simulink model "test_birdseye_transform"  (R2019a)
settings: Solver=VariableStepAuto  StartTime=0.0  StopTime=1  RelTol=1e-3
values from neighbouring files (symbols this model uses):
  T_unreal = tform.T    [estimate_birdseye_transform.m]
undefined symbols (not defined in the file or in its folder): gray, Rec, SDTV
libraries: visiongeotforms x2, visionhdlio x2, visionhdlgeotforms x1, visionconversions x1, visionsources x1, visionhdlutilities x1
settings Model: Creator=tstraessle  LastModifiedBy=timo.straessle

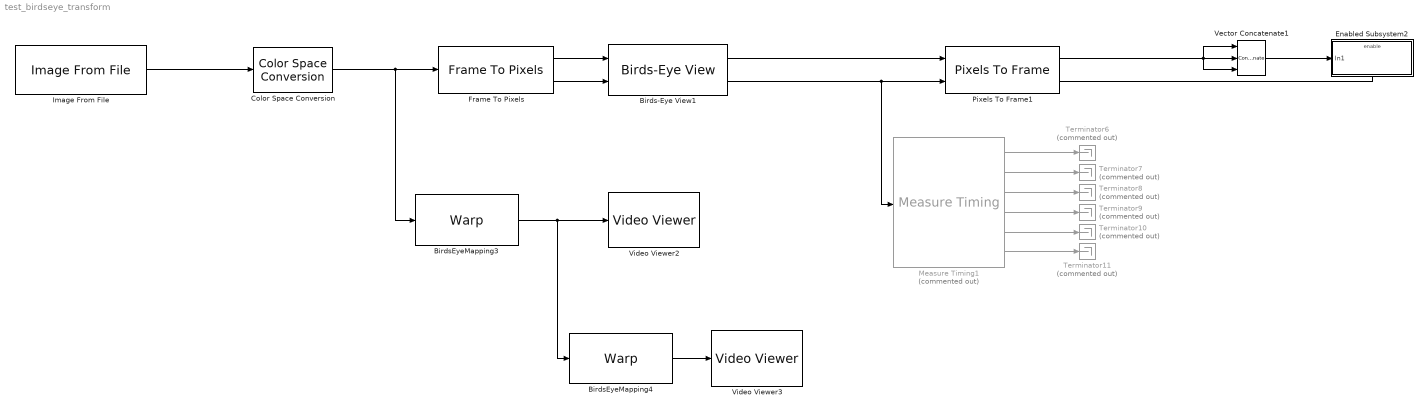
== system test_birdseye_transform ==
  Birds-Eye View1 : visionhdlgeotforms/Birds-Eye View  HomographyMatrix=T_unreal  MaxBufferSize=200000*2  MaxSourceLinesBuffered=100*2  BirdsEyeActivePixels=1920  BirdsEyeActiveLines=1080  SimulateUsing=Code generation
      settings: SourceProductName=Vision HDL Toolbox  SourceProductBaseCode=VT
  BirdsEyeMapping3 : visiongeotforms/Warp  TransformMatrixSource=Custom  TransformMatrix=T_unreal  InterpolationMethod=Bilinear  BackgroundFillValue=0  OutputImagePositionSource=Custom  OutputImagePosition=[ 1, 1, 1920, 1080 ]  ROIInputPort=off  ROIValidityOutputPort=off  SimulateUsing=Code generation
      settings: SourceProductName=Computer Vision Toolbox  SourceProductBaseCode=VP
  BirdsEyeMapping4 : visiongeotforms/Warp  TransformMatrixSource=Custom  TransformMatrix=inv(T_unreal)  InterpolationMethod=Bilinear  BackgroundFillValue=0  OutputImagePositionSource=Custom  OutputImagePosition=[ 1, 1, 1920, 1080 ]  ROIInputPort=off  ROIValidityOutputPort=off  SimulateUsing=Code generation
      settings: SourceProductName=Computer Vision Toolbox  SourceProductBaseCode=VP
  Color Space Conversion : visionconversions/Color Space  Conversion  conversion=Obsolete  conversionActive=R'G'B' to intensity  wp_str=D65  rec=Rec. 601 (SDTV)  sys=1125/60/2:1  imagePorts=One multidimensional signal
  Enabled Subsystem2 : Subsystem  TreatAsAtomicUnit=on
  Frame To Pixels : visionhdlio/Frame To Pixels  NumComponents=1  VideoFormat=1080p  ActivePixelsPerLine=1280  ActiveVideoLines=720  TotalPixelsPerLine=1650  TotalVideoLines=1100  StartingActiveLine=25  FrontPorch=110  SampleTime=0
      settings: SourceProductName=Vision HDL Toolbox  SourceProductBaseCode=VT
  Image From File : visionsources/Image From File  Tag=vipblks_nd  FileName=C:\SVN\AE\content_creation\demos\ID83 - Lane Detection on FPGA\new version\support files\images\snapshot_straight_road.bmp  Ts=1/60  imagePorts=One multidimensional signal  OutPortLabels=R|G|B  ImageDataType=uint8  sdImageDataType=uint(8)  Signed=on  WordLength=16  FractionLengthMode=User-defined  FractionLength=15
      settings: SourceProductName=Computer Vision Toolbox
  Measure Timing1 : visionhdlutilities/Measure Timing  Commented=on  SimulateUsing=Code generation
      settings: SourceProductName=Vision HDL Toolbox  SourceProductBaseCode=VT
  Pixels To Frame1 : visionhdlio/Pixels To Frame  NumComponents=1  VideoFormat=1080p  ActivePixelsPerLine=1280  ActiveVideoLines=1050  TotalPixelsPerLine=1650  TotalVideoLines=1100
      settings: SourceProductName=Vision HDL Toolbox  SourceProductBaseCode=VT
  Terminator{6..11} (6 alike) : Terminator  Commented=on
  Vector Concatenate1 : Concatenate  NumInputs=3  Mode=Multidimensional array  ConcatenateDimension=3
  Video Viewer2 : VideoViewer  colormapValue=gray(256)  FigPos=[1105 1039 769 647]
  Video Viewer3 : VideoViewer  colormapValue=gray(256)  FigPos=[1736 1117 961 767]
  wires:
  Pixels To Frame1/2 -> Enabled Subsystem2/Enable
  Vector Concatenate1/1 -> Enabled Subsystem2/1(In1)
  Pixels To Frame1/1 -> Vector Concatenate1/3, Vector Concatenate1/2, Vector Concatenate1/1
  Birds-Eye View1/1 -> Pixels To Frame1/1
  Birds-Eye View1/2 -> Measure Timing1/1, Pixels To Frame1/2
  Color Space Conversion/1 -> Frame To Pixels/1, BirdsEyeMapping3/1
  Frame To Pixels/1 -> Birds-Eye View1/1
  Frame To Pixels/2 -> Birds-Eye View1/2
  BirdsEyeMapping3/1 -> BirdsEyeMapping4/1, Video Viewer2/1
  BirdsEyeMapping4/1 -> Video Viewer3/1
  Image From File/1 -> Color Space Conversion/1
  Measure Timing1/3 -> Terminator8/1
  Measure Timing1/4 -> Terminator9/1
  Measure Timing1/2 -> Terminator7/1
  Measure Timing1/1 -> Terminator6/1
  Measure Timing1/5 -> Terminator10/1
  Measure Timing1/6 -> Terminator11/1

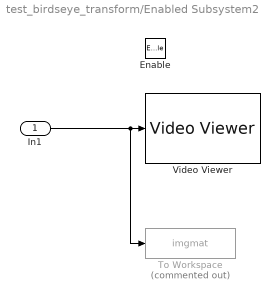
== system test_birdseye_transform/Enabled Subsystem2 ==
  In1 : Inport
  Enable : EnablePort
  To Workspace : ToWorkspace  Commented=on  VariableName=imgmat  SaveFormat=Timeseries  SampleTime=-1
  Video Viewer : VideoViewer  colormapValue=gray(256)  FigPos=[450 871 668 465]
  wires:
  In1/1 -> Video Viewer/1, To Workspace/1
